simulink model "inner_loop_outer_Geometric"  (R2019b)
settings: Solver=ode4  StartTime=0.0  StopTime=10.0  FixedStep=1e-3  RelTol=1e-3
settings Model: Creator=a5akhtar  LastModifiedBy=SamiraE
settings DataIOCC: ReturnWorkspaceOutputs=off
settings DebuggingCC: ArithmeticOperatorsInVariantConditions=warning
settings SFSimCC: CustomCodeUndefinedFunction=UseInterfaceOnly

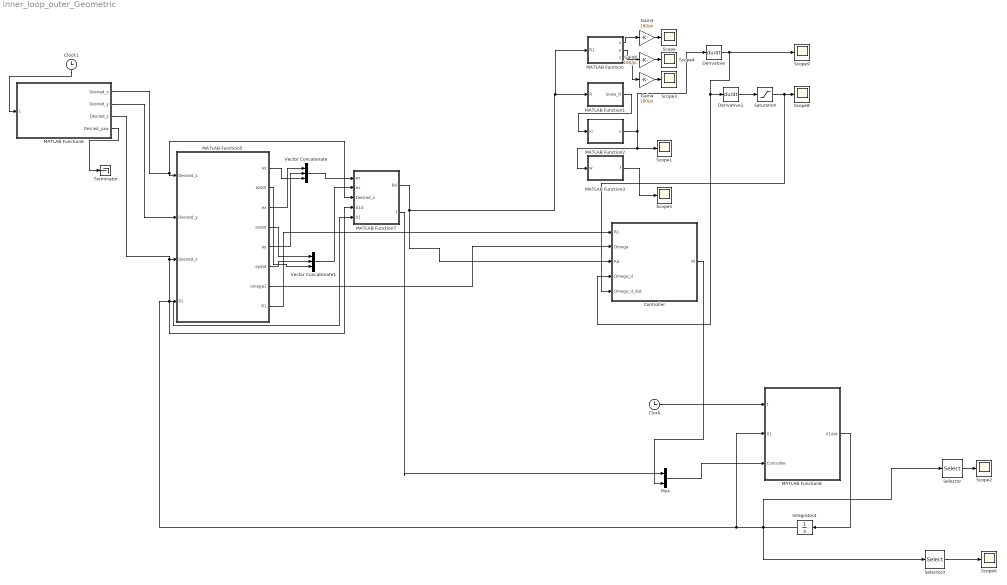
== system inner_loop_outer_Geometric ==
  Clock : Clock
  Clock1 : Clock
  Controller : MATLAB Function  TreatAsAtomicUnit=on
  Derivative : Derivative
  Derivative1 : Derivative
  Gain3 : Gain  Gain=180/pi
  Gain4 : Gain  Gain=180/pi
  Gain6 : Gain  Gain=180/pi
  Integrator4 : Integrator  InitialCondition=[0;0;0;0;0;0;reshape(eye(3),9,1);0;0;0]
  MATLAB Function : MATLAB Function  TreatAsAtomicUnit=on
  MATLAB Function1 : MATLAB Function  TreatAsAtomicUnit=on
  MATLAB Function2 : MATLAB Function  TreatAsAtomicUnit=on
  MATLAB Function3 : MATLAB Function  TreatAsAtomicUnit=on
  MATLAB Function5 : MATLAB Function  TreatAsAtomicUnit=on
  MATLAB Function6 : MATLAB Function  TreatAsAtomicUnit=on
  MATLAB Function7 : MATLAB Function  TreatAsAtomicUnit=on
  MATLAB Function8 : MATLAB Function  TreatAsAtomicUnit=on
  Mux : Mux  Inputs=2
  Saturation : Saturate  UpperLimit=20  LowerLimit=-20
  Scope{,1..6,8..9} (9 alike) : Scope
  Selector : Selector  InputPortWidth=18  IndexOptions=Index vector (dialog)  Indices=[1:2]  OutputSizes=1
  Selector3 : Selector  InputPortWidth=18  IndexOptions=Index vector (dialog)  Indices=[3]  OutputSizes=1
  Terminator : Terminator
  Vector Concatenate : Concatenate  NumInputs=3
  Vector Concatenate1 : Concatenate  NumInputs=3
  wires:
  MATLAB Function/1(x) -> Gain3/1
  MATLAB Function/2(y) -> Gain6/1
  MATLAB Function1/1(Skew_R) -> MATLAB Function2/1(xi)
  MATLAB Function2/1(v) -> Scope1/1, MATLAB Function3/1(w), Derivative/1
  MATLAB Function3/1(f) -> Scope5/1
  Derivative/1 -> Controller/4(Omega_d), Derivative1/1, Scope9/1
  Derivative1/1 -> Saturation/1
  Saturation/1 -> Controller/5(Omega_d_dot), Scope8/1
  Clock/1 -> MATLAB Function8/1(t)
  MATLAB Function5/8(R1) -> Controller/1(R1)
  Gain3/1 -> Scope/1
  Gain6/1 -> Scope4/1
  Gain4/1 -> Scope3/1
  MATLAB Function/3(z) -> Gain4/1
  Clock1/1 -> MATLAB Function6/1(t)
  MATLAB Function6/3(Desried_z) -> MATLAB Function7/4(b1d), MATLAB Function5/3(Desired_z)
  MATLAB Function6/2(Desried_y) -> MATLAB Function5/2(Desired_y)
  MATLAB Function6/1(Desried_x) -> MATLAB Function7/3(Desired_x), MATLAB Function5/1(Desired_x)
  MATLAB Function5/4(exdot) -> Vector Concatenate1/1
  MATLAB Function5/6(eydot) -> Vector Concatenate1/2
  MATLAB Function5/2(ezdot) -> Vector Concatenate1/3
  Vector Concatenate/1 -> MATLAB Function7/1(ex)
  Vector Concatenate1/1 -> MATLAB Function7/2(ev)
  MATLAB Function7/1(Rd) -> MATLAB Function/1(R1), MATLAB Function1/1(R), Controller/3(Rd)
  MATLAB Function6/4(Desried_yaw) -> Terminator/1
  MATLAB Function8/1(X1dot) -> Integrator4/1
  MATLAB Function5/7(omega1) -> Controller/2(Omega)
  MATLAB Function5/3(ex) -> Vector Concatenate/1
  MATLAB Function5/5(ey) -> Vector Concatenate/2
  MATLAB Function5/1(ez) -> Vector Concatenate/3
  MATLAB Function7/2(f) -> Mux/1
  Controller/1(M) -> Mux/2
  Mux/1 -> MATLAB Function8/3(Controller)
  Selector3/1 -> Scope6/1
  Integrator4/1 -> Selector/1, Selector3/1, MATLAB Function8/2(X1), MATLAB Function7/5(X1), MATLAB Function5/4(X1)
  Selector/1 -> Scope2/1

== matlab function inner_loop_outer_Geometric/MATLAB Function1 ==
  data: R input; Skew_R output
function Skew_R = mylogm(R)

Rp = reshape(R,3,3);
    angle = acos( (trace(Rp) - 1)/2 )
    
    if (abs(angle) == 0 )
    
    mylog = zeros(3,3);
    
    else
        mylog = (angle/(2*sin(angle)))*( Rp - Rp' );
        
    end
    
Skew_R = mylog;

== matlab function inner_loop_outer_Geometric/MATLAB Function ==
  data: x output; R1 input; y output; z output
function [x,y,z] = decompose_rotation_sim(R1)

R = reshape(R1,3,3)
	x = atan2(R(3,2), R(3,3));
	y = atan2(-R(3,1), sqrt(R(3,2)*R(3,2) + R(3,3)*R(3,3)));
	z = atan2(R(2,1), R(1,1));
end



%y = u;

== matlab function inner_loop_outer_Geometric/MATLAB Function2 ==
  data: xi input; v output
%% This function takes a 3 by 3 skew symmetric matrix and converts it into a vector.
function v = so3_hatinv(xi)
[row,col] = size(xi);

% if (row~=3 && col~=3)
%     display('dimension error! so3_hatinv only takes skew symmetric 3 by 3 matrices');
%     return;
% end
% 
% if (abs(xi(1,1))> (0.00001)  && abs(xi(2,2))> (0.00001) && abs (xi(3,3))> (0.00001))
%     display('Martix in not skew! Diagonal entries are not "zero"!!');
%     return;
% end

v = [xi(3,2); xi(1,3); xi(2,1)];
end

== matlab function inner_loop_outer_Geometric/MATLAB Function3 ==
  data: w input; f output
function f = so3_hat(w)

[row,col] = size(w);

% if (row~=3 && col~=1)
%     display('dimension error! so3_hat only takes col vectors consisting of 3 elements');
%     return;
% end

f=[0, -w(3), w(2);
   w(3), 0, -w(1);
   -w(2), w(1), 0];
end

== matlab function inner_loop_outer_Geometric/Controller ==
  data: R1 input; M output; Omega input; Rd input; Omega_d input; Omega_d_dot input
function M  = attitudeControllerSO3(R1,Omega,Rd,Omega_d,Omega_d_dot)

Jx = 0.01;
Jy = 0.0082;
Jz = 0.0148;


J = diag([Jx,Jy,Jz]);

R = reshape(R1,3,3);
R_d = reshape(Rd,3,3);

%%%%%%%%%%%%%%%%%%%%%%%%% New terms %%%%%%%%%%%%%%%%%%%%%%%%%%%%%%%%%%
    xi1 = mylogm(R'*R_d);
    V = so3_hatinv ( so3_hat(Omega) - (R'*R_d)*so3_hat(Omega_d)*(R_d'*R) ); 
    xi2 =  -so3_hat(V);
    %xi2_check =  (-so3_hat(V)*(R'*R_d))*(R'*R_d)';
    
    
    Vnew = -[50;50;50].*so3_hatinv(xi1) - [20;20;20].*so3_hatinv(xi2);
    
    U = -( Vnew );
    
    M = cross(Omega,J*Omega) + J*( U );
    

end

function Skew_R = mylogm(R)

Rp = (R);
    angle = acos( (trace(Rp) - 1)/2 )
    
    if (abs(angle) == 0 )
    
    mylog = zeros(3,3);
    
    else
        mylog = (angle/(2*sin(angle)))*( Rp - Rp' );
        
    end
    
Skew_R = mylog;
end
%% This function takes a 3 by 3 skew symmetric matrix and converts it into a vector.
function v = so3_hatinv(xi)
[row,col] = size(xi);

% if (row~=3 && col~=3)
%     display('dimension error! so3_hatinv only takes skew symmetric 3 by 3 matrices');
%     return;
% end
% 
% if (abs(xi(1,1))> (0.00001)  && abs(xi(2,2))> (0.00001) && abs (xi(3,3))> (0.00001))
%     display('Martix in not skew! Diagonal entries are not "zero"!!');
%     return;
% end

v = [xi(3,2); xi(1,3); xi(2,1)];
end
%%
function f = so3_hat(w)

[row,col] = size(w);

% if (row~=3 && col~=1)
%     display('dimension error! so3_hat only takes col vectors consisting of 3 elements');
%     return;
% end

f=[0, -w(3), w(2);
   w(3), 0, -w(1);
   -w(2), w(1), 0];
end

== matlab function inner_loop_outer_Geometric/MATLAB Function5 ==
  data: ez output; Desired_x input; Desired_y input; Desired_z input; X1 input; ezdot output; ex output; exdot output; ey output; eydot output; omega1 output; R1 output
function [ez, ezdot,ex,exdot,ey,eydot,omega1,R1] = Errors(Desired_x, Desired_y, Desired_z,X1)
%% Quadrotor
X1dot=X1;
rq=X1(1:3);
vq = X1(1+3:3+3);
R1  = X1(1+6:9+6);
omega1 = X1(9+6+1:9+6+3);

xd = Desired_x(1);
xddot = Desired_x(2);
xd2dot = Desired_x(3);
xd3dot = Desired_x(4);
xd4dot = Desired_x(5);

yd = Desired_y(1);
yddot = Desired_y(2);
yd2dot = Desired_y(3);
yd3dot = Desired_y(4);
yd4dot = Desired_y(5);

zd = Desired_z(1);
zddot = Desired_z(2);
zd2dot = Desired_z(3);
% m = 1.12;
% g=9.81;
% Jx = 0.01;
% Jy = 0.0082;
% Jz = 0.0148;
% 
% lambda1 = 1;lambda2 = 1;lambda3 = 1;lambda4 = 1;lambda5 = 1;lambda6 = 1;
% lambda7 = 1;lambda8 = 1;lambda8 = 1;lambda10 = 1;lambda11 = 1;lambda12 = 1;
% lambda13 = 1;lambda14 = 1;lambda15 = 1;lambda16 = 1;lambda17 = 1;lambda18 = 1;

ez = rq(3)-zd;
ezdot = vq(3)-zddot;
ex = rq(1)-xd;
exdot = vq(1)-xddot;
ey = rq(2)-yd;
eydot = vq(2)-yddot;
end

== matlab function inner_loop_outer_Geometric/MATLAB Function6 ==
  data: Desried_x output; t input; Desried_y output; Desried_z output; Desried_yaw output
function [Desried_x, Desried_y,Desried_z,Desried_yaw] = Desired_pose(t)
%% Quadrotor
Desried_x = [1;0;0;0;0;];

Desried_y = [1;0;0;0;0;];

Desried_z = [1;0;0;];

Desried_yaw = [0.2;0;0];
end

== matlab function inner_loop_outer_Geometric/MATLAB Function7 ==
  data: ex input; Rd output; ev input; Desired_x input; b1d input; f output; X1 input
function [Rd,f] = fcn(ex,ev,Desired_x,b1d,X1)
kx = 16;
kv = 5.6;
m = 1.14;
g = 10;

R1  = X1(1+6:9+6);
R = reshape(R1,3,3);
e3 = [0;0;1];
xd2dot = Desired_x(3);

b3d = (-kx*ex - kv*ev - m*g*e3 +m*xd2dot)/norm(-kx*ex - kv*ev - m*g*e3 +m*xd2dot);


b2d = cross(b3d,b1d)/norm(cross(b3d,b1d));

Rd = [cross(b2d,b3d); b2d; b3d];

f = -(-kx*ex - kv*ev - m*g*e3 -m*g*e3+m*xd2dot)'*R*e3;

== matlab function inner_loop_outer_Geometric/MATLAB Function8 ==
  data: t input; X1 input; X1dot output; Controller input
function X1dot   = Quadrotor_dynamics(t,X1,Controller)
%% Quadrotor
X1dot=X1;
rq=X1(1:3);
vq = X1(1+3:3+3);
R1  = X1(1+6:9+6);
omega1 = X1(9+6+1:9+6+3);

m = 1.14;
g=9.81;
Jx = 0.01;
Jy = 0.0082;
Jz = 0.0148;


 omega_i = omega1;
    
    s_omega = [0 -omega_i(3) omega_i(2);
    omega_i(3) 0 -omega_i(1);
    -omega_i(2) omega_i(1) 0];

f = Controller (1);

X1dot(1:3) = vq;
X1dot(4:6) = -m*g*[0;0;1] +f *reshape(R1,3,3)*[0;0;1];
X1dot(1+6:9+6) = reshape(reshape(R1,3,3)*s_omega,9,1);
X1dot(9+6+1:9+6+3) = diag([Jx,Jy,Jz])\( - s_omega*diag([Jx,Jy,Jz])*omega_i+Controller(2:4));

end
